simulink model "reduced_7_lvl"  (R2023a)
settings: Solver=ode45  StartTime=0.0  StopTime=0.2  RelTol=1e-3  EnableMultiTasking=on
libraries: simulink x6, spsMosfetLib x5, spsDCVoltageSourceLib x4, spsCurrentMeasurementLib x1, spsGroundLib x1, spsSeriesRLCBranchLib x1, spsVoltageMeasurementLib x1, spspowerguiLib x1
settings Model: Creator=R.K.Kumawat  LastModifiedBy=dhana
settings SolverCC: AlgebraicLoopSolver=TrustRegion
settings DataIOCC: LimitDataPoints=on  SaveFormat=Array  SignalLoggingSaveFormat=ModelDataLogs  ReturnWorkspaceOutputs=off
settings OptimizationCC: ExpressionDepthLimit=2147483647  LifeSpan=inf
settings DebuggingCC: UnderspecifiedInitializationDetection=Classic  MergeDetectMultiDrivingBlocksExec=none  SolverPrmCheckMsg=warning  FcnCallInpInsideContextMsg=warning  UnconnectedInputMsg=warning  UnconnectedOutputMsg=warning  UnconnectedLineMsg=warning  StateNameClashWarn=warning  SFUnexpectedBacktrackingDiag=warning  SFNoUnconditionalDefaultTransitionDiag=warning  SFExecutionAtInitializationDiag=none  ArithmeticOperatorsInVariantConditions=warning
settings HardwareCC: ProdBitPerPointer=32  ProdBitPerSizeT=32  ProdBitPerPtrDiffT=32  ProdLargestAtomicFloat=None  ProdIntDivRoundTo=Undefined  ProdEndianess=Unspecified  ProdWordSize=32  ProdHWDeviceType=32-bit Generic
settings ModelReferenceCC: PropagateSignalLabelsOutOfModel=off
settings SFSimCC: SimUseLocalCustomCode=off  CustomCodeUndefinedFunction=UseInterfaceOnly
settings RTWCC: RTWUseLocalCustomCode=off
settings CodeAppCC: StateflowObjectComments=on
settings GRTTargetCC: TargetLangStandard=C89/C90 (ANSI)
settings ConfigComp: CovMetricSettings=dw  CovSaveCumulativeToWorkspaceVar=on  CovSaveSingleToWorkspaceVar=on  CovExternalEMLEnable=off
settings SimscapeCC: SimscapeNormalizeSystem=off

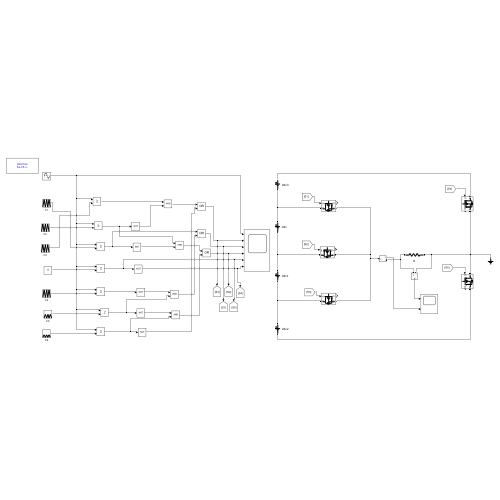
[thumbnail: Simulink's stored preview of the top-level diagram]
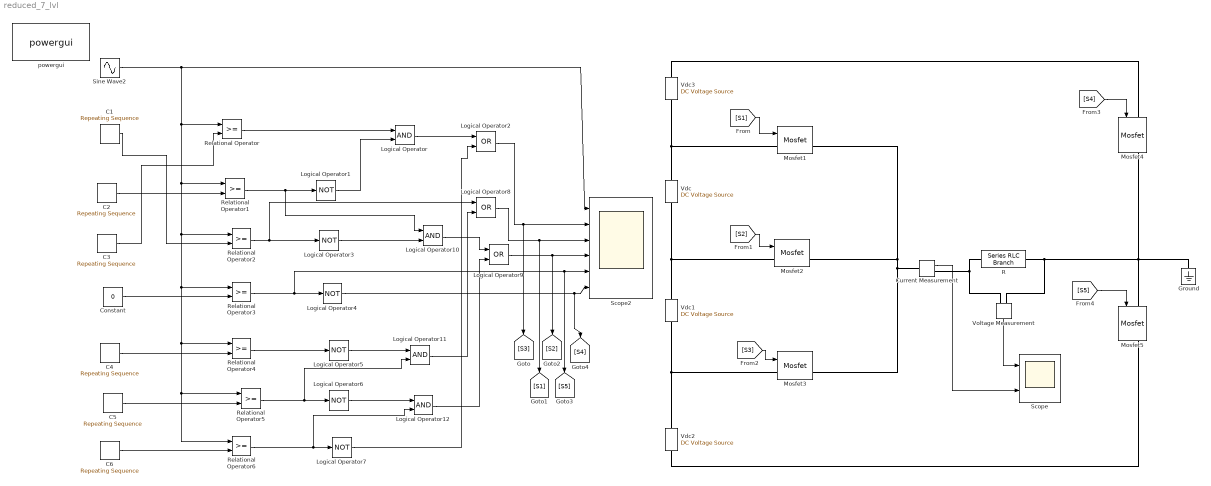
== system reduced_7_lvl ==
  C1 : simulink/Sources/Repeating Sequence  rep_seq_t=[0 1/10000 1/5000]  rep_seq_y=[4 6 4]
  C2 : simulink/Sources/Repeating Sequence  rep_seq_t=[0 1/10000 1/5000]  rep_seq_y=[2 4 2]
  C3 : simulink/Sources/Repeating Sequence  rep_seq_t=[0 1/10000 1/5000]  rep_seq_y=[0 2 0]
  C4 : simulink/Sources/Repeating Sequence  rep_seq_t=[0 1/10000 1/5000]  rep_seq_y=[-2 0 -2]
  C5 : simulink/Sources/Repeating Sequence  rep_seq_t=[0 1/10000 1/5000]  rep_seq_y=[-4 -2 -4]
  C6 : simulink/Sources/Repeating Sequence  rep_seq_t=[0 1/10000 1/5000]  rep_seq_y=[-6 -4 -6]
  Constant : Constant  Value=0
  Current Measurement : spsCurrentMeasurementLib/Current Measurement  PhasorSimulation=off  OutputType=Complex  PSBequivalent=0
  Ground : spsGroundLib/Ground  LConnTagsString=a
  Logical Operator{,10..12} (4 alike) : Logic  AllPortsSameDT=off  OutDataTypeStr=boolean
  Logical Operator{1,3..7} (6 alike) : Logic  Operator=NOT  AllPortsSameDT=off  OutDataTypeStr=boolean
  Logical Operator2 : Logic  Operator=OR  AllPortsSameDT=off  OutDataTypeStr=boolean
  Logical Operator8 : Logic  Operator=OR  AllPortsSameDT=off  OutDataTypeStr=boolean
  Logical Operator9 : Logic  Operator=OR  AllPortsSameDT=off  OutDataTypeStr=boolean
  Mosfet{1..5} (5 alike) : spsMosfetLib/Mosfet  Ron=0.01  Lon=0  Rd=10000  Vfd=0  IC=0  Rs=1e5  Cs=inf  Measurements=on
  R : spsSeriesRLCBranchLib/Series RLC Branch  LConnTagsString=__new0  RConnTagsString=__new0  BranchType=R  Resistance=10  Inductance=1e-3  SetiL0=off  InitialCurrent=0  Capacitance=1e-6  Setx0=off  InitialVoltage=0  Measurements=None
  Relational Operator{,1..6} (7 alike) : RelationalOperator  OutDataTypeStr=boolean  InputSameDT=off
  Scope : Scope  NumInputPorts=2
  Scope2 : Scope  NumInputPorts=6
  Sine Wave2 : Sin  Amplitude=6  Frequency=2*pi*50  SampleTime=1e-6
  Vdc{,1..3} (4 alike) : spsDCVoltageSourceLib/DC Voltage Source  Amplitude=100  Measurements=None
  Voltage Measurement : spsVoltageMeasurementLib/Voltage Measurement  PhasorSimulation=off  OutputType=Complex  PSBequivalent=0
  powergui : spspowerguiLib/powergui  Priority=1  SimulationMode=Discrete  SampleTime=5e-005  frequency=60  Iterations=50  frequencyindice=0  Pbase=100e6  ErrMax=1e-4  UnitsV=kV  UnitsW=MW  buscounter=0  FunctionMessages=off  echomessages=off  EnableUseOfTLC=off  CurrentSourceSwitches=off  DisableSnubberDevices=off  DisableRonSwitches=off  DisableVfSwitches=off  DisplayEquations=off  AutomaticDiscreteSolvers=off  SolverType=Tustin  Interpol=off  ExternalGateDelay=off  methode=off  Ts=100  x0status=blocks  SPID=off  SwTol=0  HookPort=off  NonlinearTolerance=1e-4  nMaxIteration=100  ContinueOnMaxIteration=off  RestoreLinks=warning  ResistiveCurrentMeasurement=off  Frange=[0:2:500]  Ylog=off  Xlog=on  ShowGrid=off  save=off  variable=ZData  structure=0  ZoomFFT=off  StartTime=0.0  cycles=1  DisplayStyle=1  fundamental=60  FreqAxis=off  MaxFrequency=1000  frequencyindicesteady=1  RmsSteady=1  display=off
  wires:
  Sine Wave2/1 -> Scope2/1, Relational Operator/1, Relational Operator1/1, Relational Operator2/1, Relational Operator3/1, Relational Operator4/1, Relational Operator5/1, Relational Operator6/1
  C2/1 -> Relational Operator1/2
  Constant/1 -> Relational Operator3/2
  C4/1 -> Relational Operator4/2
  C5/1 -> Relational Operator5/2
  C6/1 -> Relational Operator6/2
  Relational Operator/1 -> Logical Operator/1
  Relational Operator1/1 -> Logical Operator1/1, Logical Operator10/1
  Logical Operator1/1 -> Logical Operator/2
  Logical Operator/1 -> Logical Operator2/1
  Relational Operator2/1 -> Logical Operator8/1, Logical Operator3/1
  Relational Operator3/1 -> Logical Operator4/1, Scope2/5, [S5]
  Relational Operator4/1 -> Logical Operator5/1
  Relational Operator5/1 -> Logical Operator6/1, Logical Operator11/2
  Relational Operator6/1 -> Logical Operator7/1, Logical Operator12/2
  Logical Operator3/1 -> Logical Operator10/2
  Logical Operator7/1 -> Logical Operator2/2
  Logical Operator5/1 -> Logical Operator11/1
  Logical Operator11/1 -> Logical Operator8/2
  Logical Operator10/1 -> Logical Operator9/1
  Logical Operator6/1 -> Logical Operator12/1
  Logical Operator12/1 -> Logical Operator9/2
  Logical Operator4/1 -> Scope2/6, [S4]
  Logical Operator2/1 -> Scope2/2, [S3]
  Logical Operator8/1 -> Scope2/3, [S1]
  Logical Operator9/1 -> Scope2/4, [S2]
  [S1] -> Mosfet1/1
  [S2] -> Mosfet2/1
  [S3] -> Mosfet3/1
  [S4] -> Mosfet4/1
  [S5] -> Mosfet5/1
  Voltage Measurement/1 -> Scope/1
  C3/1 -> Relational Operator/2
  C1/1 -> Relational Operator2/2
  Current Measurement/1 -> Scope/2
  connections:
  Mosfet2/LConn1 -- Vdc/LConn1 -- Vdc1/RConn1
  Mosfet3/LConn1 -- Vdc2/RConn1 -- Vdc1/LConn1
  Mosfet1/LConn1 -- Vdc3/LConn1 -- Vdc/RConn1
  Voltage Measurement/LConn1 -- Current Measurement/RConn1 -- R/LConn1
  Voltage Measurement/LConn2 -- Mosfet4/RConn1 -- Mosfet5/LConn1 -- Ground/LConn1 -- R/RConn1
  Vdc2/LConn1 -- Mosfet5/RConn1
  Vdc3/RConn1 -- Mosfet4/LConn1
  Mosfet1/RConn1 -- Current Measurement/LConn1 -- Mosfet3/RConn1 -- Mosfet2/RConn1
